simulink model "Assignment2_3"  (R2020a)
settings: Solver=FixedStepAuto  StartTime=0.0  StopTime=10.0  FixedStep=1e-3  RelTol=1e-3  EnableMultiTasking=on
undefined symbols (not defined in the file or in its folder): D10, D11, D12, D2, D4, D5, D7, D8, D9, PTA0, PTA2, PTB23, PTB9, PTC3, PTC4, PTD0, PTD2, PTD3
libraries: frdmk64flib x9
settings Model: ExtModeTrigDuration=5  Creator=iceca  LastModifiedBy=iceca
settings OptimizationCC: EnhancedBackFolding=on  PassReuseOutputArgsAs=Individual arguments  ZeroExternalMemoryAtStartup=off  ZeroInternalMemoryAtStartup=off  MaxStackSize=64  OptimizeBlockOrder=speed  DifferentSizesBufferReuse=on  OptimizationCustomize=off  EfficientTunableParamExpr=on
settings DebuggingCC: ParameterTunabilityLossMsg=error
settings HardwareCC: ProdBitPerPointer=32  ProdBitPerSizeT=32  ProdBitPerPtrDiffT=32  ProdLargestAtomicInteger=Long  ProdLargestAtomicFloat=Double  ProdWordSize=32  ProdHWDeviceType=ARM Compatible->ARM Cortex
settings SFSimCC: MATLABDynamicMemAlloc=off
settings RTWCC: SystemTargetFile=ert.tlc  HardwareBoard=NXP FRDM-K64F  TemplateMakefile=ert_default_tmf  Toolchain=GNU Tools for ARM Embedded Processors
settings CodeAppCC: ForceParamTrailComments=on  IgnoreCustomStorageClasses=off  OperatorAnnotations=on  SimulinkDataObjDesc=on  SFDataObjDesc=on  InsertBlockDesc=on

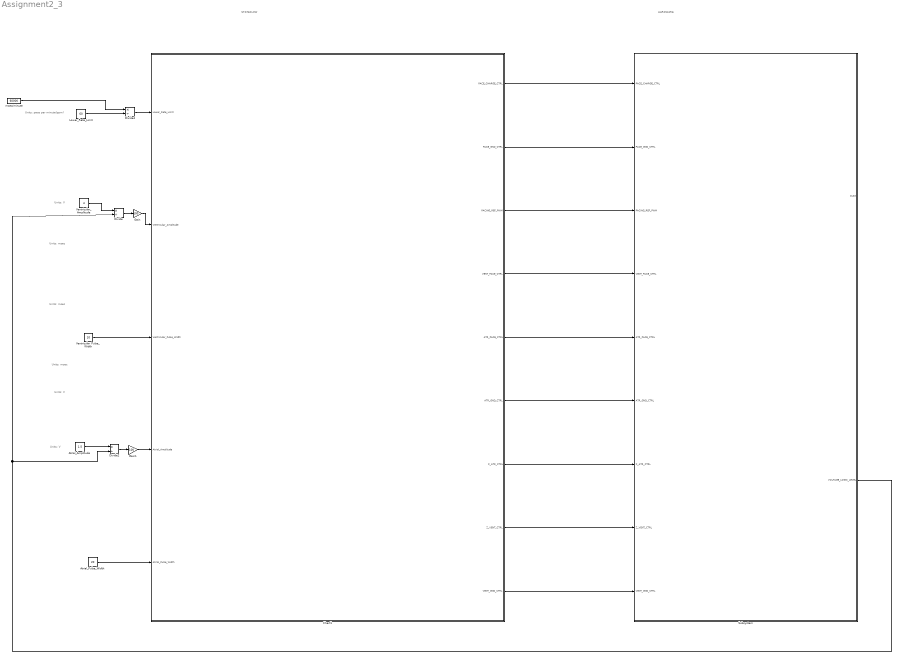
== system Assignment2_3 ==
  note: Units: pace per minute(ppm)
  note: HARDWARE
  note: Units: V
  note: Units: V
  note: Units: msec
  note: Units: msec
  note: Units: V
  note: STATEFLOW
  note: Units: msec
  Atrial_Amplitude : Constant  Value=1.5
  Atrial_Pulse_Width : Constant  Value=20
  Chart1 : Stateflow chart  TreatAsAtomicUnit=on
  Divide : Product  Inputs=*/
  Divide2 : Product  Inputs=*/
  Divide4 : Product  Inputs=*/
  Gain : Gain  Gain=100
  Gain1 : Gain  Gain=100
  Lower_Rate_Limit : Constant  Value=60
  Subsystem : Subsystem
  Ventricular_Amplitude : Constant  Value=4
  Ventricular_Pulse_Width : Constant  Value=10
  msec/minute : Constant  Value=60000
  wires:
  Divide4/1 -> Chart1/1(Lower_Rate_Limit)
  Atrial_Pulse_Width/1 -> Chart1/5(Atrial_Pulse_Width)
  Chart1/5(ATR_PACE_CTRL) -> Subsystem/5(ATR_PACE_CTRL)
  Chart1/7(Z_ATR_CTRL) -> Subsystem/7(Z_ATR_CTRL)
  Chart1/6(ATR_GND_CTRL) -> Subsystem/6(ATR_GND_CTRL)
  Chart1/9(VENT_GND_CTRL) -> Subsystem/9(VENT_GND_CTRL)
  Lower_Rate_Limit/1 -> Divide4/2
  Gain1/1 -> Chart1/4(Atrial_Amplitude)
  Chart1/2(PACE_GND_CTRL) -> Subsystem/2(PACE_GND_CTRL)
  msec/minute/1 -> Divide4/1
  Chart1/4(VENT_PACE_CTRL) -> Subsystem/4(VENT_PACE_CTRL)
  Gain/1 -> Chart1/2(Ventricular_Amplitude)
  Divide/1 -> Gain/1
  Ventricular_Pulse_Width/1 -> Chart1/3(Ventricular_Pulse_Width)
  Chart1/1(PACE_CHARGE_CTRL) -> Subsystem/1(PACE_CHARGE_CTRL)
  Chart1/3(PACING_REF_PWM) -> Subsystem/3(PACING_REF_PWM)
  Subsystem/2(VOLTAGE_LOGIC_LEVEL) -> Divide/2, Divide2/2
  Divide2/1 -> Gain1/1
  Atrial_Amplitude/1 -> Divide2/1
  Chart1/8(Z_VENT_CTRL) -> Subsystem/8(Z_VENT_CTRL)
  Ventricular_Amplitude/1 -> Divide/1

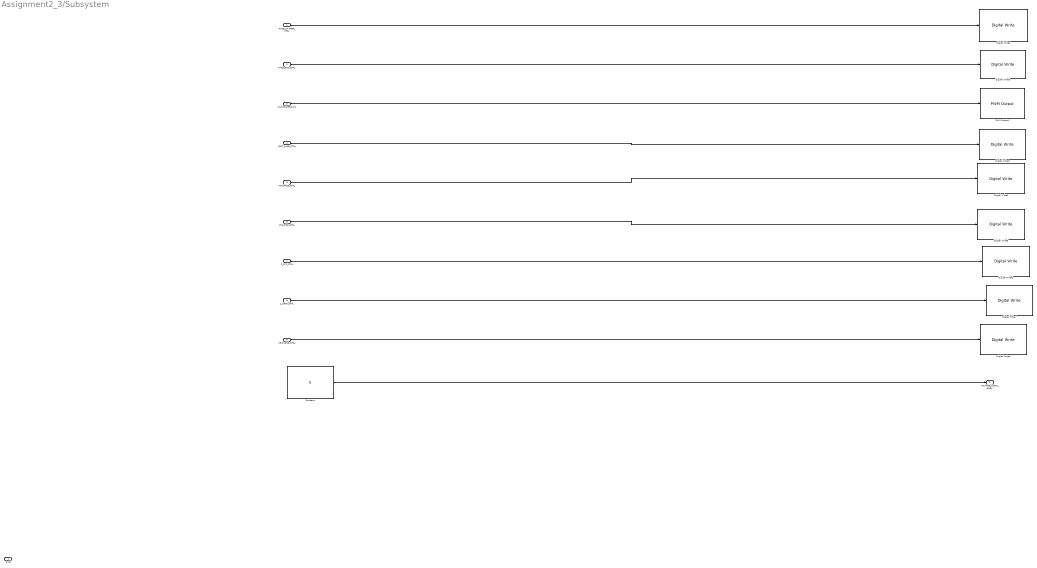
== system Assignment2_3/Subsystem ==
  PACE_CHARGE_CTRL : Inport
  PACE_GND_CTRL : Inport  Port=2
  PACING_REF_PWM : Inport  Port=3
  VENT_PACE_CTRL : Inport  Port=4
  ATR_PACE_CTRL : Inport  Port=5
  ATR_GND_CTRL : Inport  Port=6
  Z_ATR_CTRL : Inport  Port=7
  Z_VENT_CTRL : Inport  Port=8
  VENT_GND_CTRL : Inport  Port=9
  Constant : Constant  Value=5
  Digital Write2 : frdmk64flib/Digital Write  Whichpin=PTB9 (D2)
  Digital Write3 : frdmk64flib/Digital Write  Whichpin=PTD0 (D10)
  Digital Write4 : frdmk64flib/Digital Write  Whichpin=PTA0 (D8)
  Digital Write5 : frdmk64flib/Digital Write  Whichpin=PTD2 (D11)
  Digital Write6 : frdmk64flib/Digital Write  Whichpin=PTB23 (D4)
  Digital Write7 : frdmk64flib/Digital Write  Whichpin=PTC3 (D7)
  Digital Write8 : frdmk64flib/Digital Write  Whichpin=PTC4 (D9)
  Digital Write9 : frdmk64flib/Digital Write  Whichpin=PTD3 (D12)
  PWM Output1 : frdmk64flib/PWM Output  Whichpin=PTA2 (D5)  InitialFrequency=2000  InitialDutyCycle=0
  Out3 : Outport
  VOLTAGE_LOGIC_LEVEL : Outport  Port=2
  wires:
  PACING_REF_PWM/1 -> PWM Output1/1
  VENT_GND_CTRL/1 -> Digital Write9/1
  PACE_GND_CTRL/1 -> Digital Write3/1
  ATR_GND_CTRL/1 -> Digital Write5/1
  VENT_PACE_CTRL/1 -> Digital Write8/1
  Z_VENT_CTRL/1 -> Digital Write7/1
  Z_ATR_CTRL/1 -> Digital Write6/1
  PACE_CHARGE_CTRL/1 -> Digital Write2/1
  ATR_PACE_CTRL/1 -> Digital Write4/1
  Constant/1 -> VOLTAGE_LOGIC_LEVEL/1

== stateflow chart Assignment2_3/Chart1 ==
  state Charging_C22
    entry:
    ATR_PACE_CTRL   = LOW;
    VENT_PACE_CTRL = LOW;
  state Charging_C23
    entry:
    ATR_PACE_CTRL   = LOW;
    VENT_PACE_CTRL = LOW;
  state Atrial_Charge
    entry:
    PACING_REF_PWM = Atrial_Amplitude;
  state Ventricular_Charge
    entry:
    PACING_REF_PWM = Ventricular_Amplitude;
  state Discharging_C21_and_Pace_Interval_Calculations1
    entry:
    PACE_CHARGE_CTRL = HIGH;
    %Discharging C21
    PACE_GND_CTRL=HIGH;
    VENT_PACE_CTRL=LOW;
    Z_ATR_CTRL= LOW;
    Z_VENT_CTRL = LOW;
    ATR_PACE_CTRL = LOW;
    Pace_Interval = Lower_Rate_Limit;
  state Discharging_C21_and_Pace_Interval_Calculations
    entry:
    PACE_CHARGE_CTRL = HIGH;
    %Discharging C21
    PACE_GND_CTRL=HIGH;
    VENT_PACE_CTRL=LOW;
    Z_ATR_CTRL= LOW;
    Z_VENT_CTRL = LOW;
    ATR_PACE_CTRL = LOW;
    Pace_Interval = Lower_Rate_Limit;
  state Atrial_Discharge
    entry:
    ATR_GND_CTRL= HIGH;
    VENT_GND_CTRL= LOW;
    Pace_Interval =Pace_Interval-Atrial_Pulse_Width;
  state Ventricular_Discharge
    entry:
    ATR_GND_CTRL = LOW;
    VENT_GND_CTRL = HIGH;
    Pace_Interval =Pace_Interval -Ventricular_Pulse_Width;
  state No_Natural_Activity_Sensed
  state No_Natural_Activity_Sensed1
  state Pacing_Begin
    entry:
    PACE_CHARGE_CTRL = LOW;
    PACE_GND_CTRL = HIGH;
  state Pacing_Begin1
    entry:
    PACE_CHARGE_CTRL = LOW;
    PACE_GND_CTRL = HIGH;
  state Ventricular_Pacing
    entry:
    ATR_PACE_CTRL = LOW;
  state Atrial_Pacing
    entry:
    VENT_PACE_CTRL = LOW;
  state Pacing
    entry:
    ATR_GND_CTRL =LOW;
    Z_ATR_CTRL = LOW;
    Z_VENT_CTRL = LOW;
    VENT_GND_CTRL = LOW;
  state Pacing1
    entry:
    ATR_GND_CTRL =LOW;
    Z_ATR_CTRL = LOW;
    Z_VENT_CTRL = LOW;
    VENT_GND_CTRL = LOW;
  state Vent_Pacing_2
    entry:
    VENT_PACE_CTRL =HIGH;
  state Atrial_Pacing_2
    entry:
    ATR_PACE_CTRL =HIGH;
  Vent_Pacing_2 -> Charging_C22 : [after(Ventricular_Pulse_Width,msec)]
  (default) -> Charging_C23
  Atrial_Pacing_2 -> Charging_C23 : [after(Atrial_Pulse_Width,msec)]
  Charging_C23 -> Atrial_Charge
  Charging_C22 -> Ventricular_Charge
  Atrial_Charge -> Discharging_C21_and_Pace_Interval_Calculations1
  Ventricular_Charge -> Discharging_C21_and_Pace_Interval_Calculations
  Discharging_C21_and_Pace_Interval_Calculations1 -> Atrial_Discharge
  Discharging_C21_and_Pace_Interval_Calculations -> Ventricular_Discharge
  Atrial_Discharge -> No_Natural_Activity_Sensed1 : [after(Pace_Interval, msec)]
  Ventricular_Discharge -> No_Natural_Activity_Sensed : [after(Pace_Interval, msec)]
  No_Natural_Activity_Sensed -> Pacing_Begin
  No_Natural_Activity_Sensed1 -> Pacing_Begin1
  Pacing_Begin -> Ventricular_Pacing
  Pacing_Begin1 -> Atrial_Pacing
  Ventricular_Pacing -> Pacing
  Atrial_Pacing -> Pacing1
  Pacing -> Vent_Pacing_2
  Pacing1 -> Atrial_Pacing_2
  data: PACE_CHARGE_CTRL output; PACE_GND_CTRL output; PACING_REF_PWM output; VENT_PACE_CTRL output; ATR_PACE_CTRL output; ATR_GND_CTRL output; Z_ATR_CTRL output; Z_VENT_CTRL output; VENT_GND_CTRL output; Lower_Rate_Limit input; HIGH local boolean =true; LOW local boolean =false; Ventricular_Amplitude input; Ventricular_Pulse_Width input; Atrial_Amplitude input; Atrial_Pulse_Width input; Pace_Interval local
